simulink model "test"  (R2025b)
settings: Solver=VariableStepAuto  StartTime=0.0  StopTime=1  RelTol=1e-3
undefined symbols (not defined in the file): PL_frame_size, Ts
libraries: commrfcorlib x1, commfilt2 x1, dspsrcs4 x1, commsync2 x1
settings Model: Creator=Djaga  LastModifiedBy=Djaga
settings OptimizationCC: ZeroExternalMemoryAtStartup=off  ZeroInternalMemoryAtStartup=off
settings SFSimCC: SimCustomHeaderCode=pldescrambler.h  SimUserIncludeDirs=../cpp  SimUserLibraries=dvbs2.dll  SimTargetLang=C++
settings RTWCC: TargetLang=C++
settings GRTTargetCC: TargetLangStandard=C++11 (ISO)  CodeInterfacePackaging=C++ class  SubcomponentCodeInterfacePackaging=C++ class

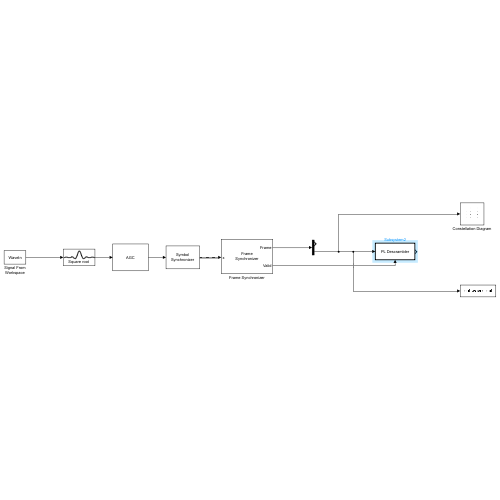
[thumbnail: Simulink's stored preview of the top-level diagram]
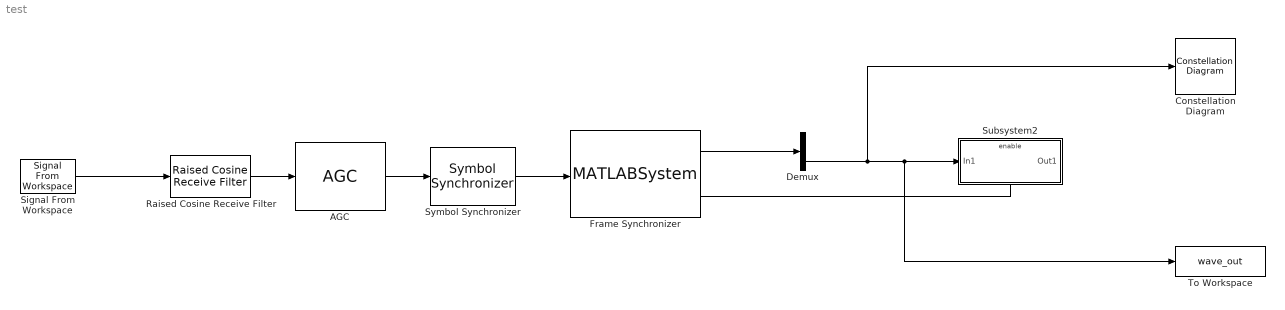
== system test ==
  AGC : commrfcorlib/AGC  LegacyMode=off  DetectorMethod=Rectifier  LoopMethod=Linear  UpdatePeriod=100  StepSize=0.1  AdaptationStepSize=0.01  DesiredOutputPower=1  AveragingLength=100  MaximumGain=30  MaxPowerGain=60  GainOutputPort=off  InputPowerOutputPort=off  SimulateUsing=Interpreted execution
  Constellation Diagram : ConstellationDiagram  WindowPosition=[1253.000000,190.000000,602.000000,517.000000,]  Visible=on  ScopeFrameLocation=window  SymbolsToDisplaySource=Property  SymbolsToDisplay=1000  ReferenceConstellation="[0.70711+0.70711i        -0.70711+0.70711i        -0.70711-0.70711i         0.70711-0.70711i]"  ShowLegend=on  MeasurementInterval=1000
  Demux : Demux  Outputs=[90, 33192]
  Frame Synchronizer : MATLABSystem  System=FrameSynchronizer  Preamble=SOF  Threshold=6  OutputLength=PL_frame_size  SimulateUsing=Interpreted execution
      mask Type: FrameSynchronizer
  Raised Cosine Receive Filter : commfilt2/Raised Cosine Receive Filter  filtType=Square root  R=0.35  filtSpan=10  N=4  downFactor=2  downOffset=0  filterGain=1  InputProcessing=Columns as channels (frame based)  RateOptions=Enforce single-rate processing  framing=Mute  checkCoeff=off  variableName=rcRxFilt  currentFiltSpan=10  D=5  inputOffset=0  sampMode=Mute  saveAsFlag=0  rateMode=Downsampling  checkGain=Normalized  launchFVT=on  roundingMode=Floor  overflowMode=off  coeffDataTypeStr=Inherit: Same word length as input  coeffMin=[]  coeffMax=[]  coeffLastDataTypeStr=Inherit: Same word length as input  accumDataTypeStr=Inherit: Same as product output  accumLastDataTypeStr=Inherit: Same as product output  outputDataTypeStr=Inherit: Same as accumulator  outputMin=[]  outputMax=[]  outputLastDataTypeStr=Inherit: Same as accumulator
  Signal From Workspace : dspsrcs4/Signal From Workspace  X=WaveIn  Ts=6016 * Ts / 133128  nsamps=133128  OutputAfterFinalValue=Setting to zero  ignoreOrWarnInputAndFrameLengths=off  OutputFrames=off
  Subsystem2 : Subsystem
      mask Display: disp('PL Descrambler');
  Symbol Synchronizer : commsync2/Symbol Synchronizer  Modulation=PAM/PSK/QAM  TimingErrorDetector=Gardner (non-data-aided)  SamplesPerSymbol=2  DampingFactor=1  NormalizedLoopBandwidth=0.01  DetectorGain=2.7  TimingErrorOutputPort=off  SimulateUsing=Code generation
  To Workspace : ToWorkspace  VariableName=wave_out  SampleTime=-1
      settings: Save2DSignal=2-D array (concatenate along first dimension)
  wires:
  AGC/1 -> Symbol Synchronizer/1
  Symbol Synchronizer/1 -> Frame Synchronizer/1
  Raised Cosine Receive Filter/1 -> AGC/1
  Frame Synchronizer/2 -> Subsystem2/Enable
  Signal From Workspace/1 -> Raised Cosine Receive Filter/1
  Frame Synchronizer/1 -> Demux/1
  Demux/2 -> Constellation Diagram/1, To Workspace/1, Subsystem2/1(In1)

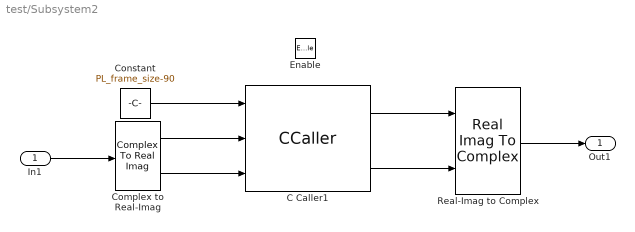
== system test/Subsystem2 ==
  In1 : Inport
  Enable : EnablePort  StatesWhenEnabling=reset
  C Caller1 : CCaller  FunctionName=pldescrambler  PortSpecificationStruct="%)30     .    * D   8    (     @         %    \"     4    !     0         %  0 \"0    $    _    07)G3F%M90  4&]R=$YA;64 4V-O<&4     26YD97@     5'EP90      4VEZ90      27-';&]B86P   X   !(    !@    @    $          4    (     0   !8    !         !     6    9G)A;65?<VEZ95]W:71H;W5T7U!,4P  #@   $@    &    \"     0         !0    @    !    %@    $         $    !8   !F<F%M95]S:7IE7W=I=&AO=71?4$Q3   .    ...(+2772 chars)"
  Complex to Real-Imag : ComplexToRealImag
  Constant : Constant  Value=PL_frame_size-90  VectorParams1D=off  OutDataTypeStr=int32
  Real-Imag to Complex : RealImagToComplex
  Out1 : Outport
  wires:
  In1/1 -> Complex to Real-Imag/1
  Real-Imag to Complex/1 -> Out1/1
  C Caller1/2 -> Real-Imag to Complex/2
  C Caller1/1 -> Real-Imag to Complex/1
  Constant/1 -> C Caller1/1
  Complex to Real-Imag/1 -> C Caller1/2
  Complex to Real-Imag/2 -> C Caller1/3
